simulink model "mcs_ut"  (Simulink 8.1)
settings: Solver=FixedStepDiscrete  StartTime=0.0  StopTime=Inf  FixedStep=0.005  RelTol=1e-3
PostLoadFcn:
  | , if any(exist('dsrtsu_mdlpostloadfcn', 'file') == [2, 3, 6]), try dsrtsu_mdlpostloadfcn('Execute', bdroot); catch fprintf('Error in PostLoadFcn (dsrtsu_mdlpostloadfcn) for model "%s":\n %s\n', bdroot, lasterr); end, end,
libraries: siltestlib x28, idiada_lib x17, mcs x1
settings Model: DSRTSU_INTERNAL_RTI_VER=450  DSRTSU_INTERNAL_RTI_TYPE=rti1401  RTICANMMDATA=struct('GeneralSetupData',struct('modelroot','D:\ELN150201_TAIWAN\trunk\AdasDragon\software\sw_development\arch\app\ifo','generalsettings',struct('filesettings',struct('destfolder',struct('Name','RTICANMM_FILES','Check',1),'buildfolder',struct('Name','.','Check',1),'AbsDestfolder',struct('Name','D:\ELN150201_TAIWAN\trunk\AdasDragon\software\sw_development\arch\app\ifo\RTICANMM_FILES'),'AbsBuildfolder',struct('Name','D:\ELN150201_TAIWAN\trunk\AdasDragon\software\sw_development\arch\app\ifo'))),'options',struct('addpaths',1,'rmpaths',1,'addtrcexclusion',logical(1),'cannavigator',struct('checkmonitoring',0),'show_usrtrc',0,'use_usrtrc',0),'advanced',struct('options',[1 1 1 1 1 1 1 1 1 1 1 1 1 1 1 1 1 1 1 1 1 1 1 1 1 1 1 1 1 1 1 1 1 1 1 1 1 1 1 1 1 1 1 1 1 1 1 1 1 1 1 1 1 1 1 1 1 1 1 1 1 1 1 1 1 1 1 1 1 1 1 1 1 1 1 1 1 1 1 1 1 1 1 1 1 1 1 1 1 1 1 1 1 1 1 1 1 1 1 1]),'MPSetup',{{}},'modelname','mcs_ut','block','mcs_ut'))  DSRTSU_INTERNAL_RTIFPGA=40  Creator=tescamilla  LastModifiedBy=AT015555  BufferReuse=off
settings DataIOCC: SignalLoggingSaveFormat=Dataset
settings OptimizationCC: BlockReduction=off  OptimizeBlockIOStorage=off  BufferReuse=off  ExpressionFolding=off  ExpressionDepthLimit=128  LocalBlockOutputs=off
settings DebuggingCC: FcnCallInpInsideContextMsg=EnableAllAsError
settings HardwareCC: ProdIntDivRoundTo=Zero  ProdEndianess=BigEndian  ProdHWDeviceType=Generic->Custom  TargetIntDivRoundTo=Zero  TargetEndianess=BigEndian  TargetHWDeviceType=Generic->Custom
settings RTWCC: SystemTargetFile=rti1401.tlc  MakeCommand=make_rti  TemplateMakefile=rti1401.tmf  Description=dSPACE DS1401 Hardware Platform  ProcessScript=rti1401_make_rtw_hook
settings STFCustomTargetCC: CodeReplacementLibrary=ANSI_C  ParMdlRefBuildCompliant=on  GeneratePreprocessorConditionals=Disable all  MatFileLogging=on  SystemTargetFile=rti1401.tlc
settings GRTTargetCC: CompOptLevelCompliant=off  ConcurrentExecutionCompliant=off  ExtModeMexFile=noextcomm
settings CustomProperty: DataType=RTWOptions_EnumType_C__Program Files (x86)_dSPACE RCPHIL 2014-B_MATLAB_RTI_RTI1401_TLC_rti1401_1InitialSimState  Value=RUN
settings EnumStrPairs: String=RUN

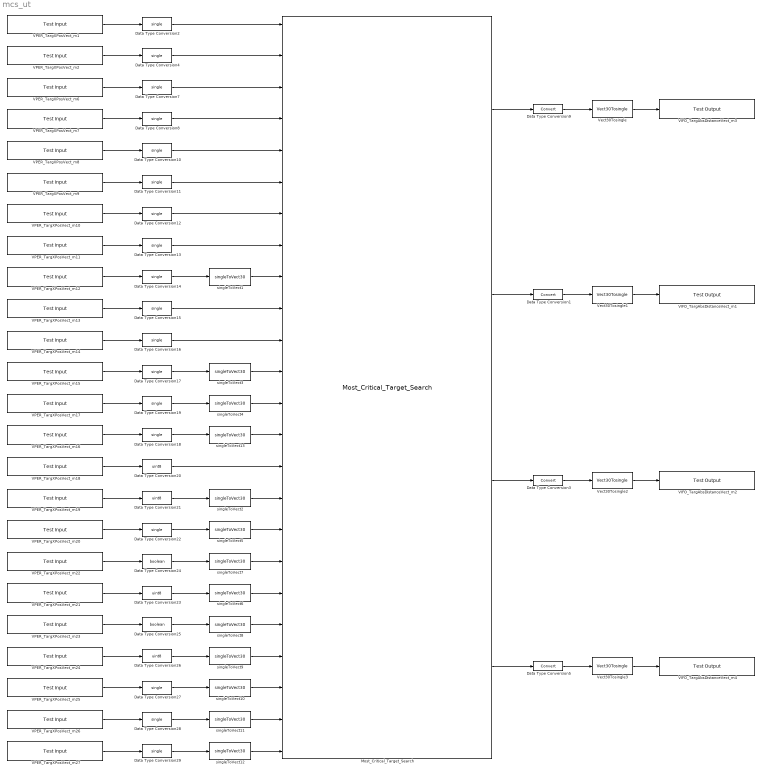
== system mcs_ut ==
  Data Type Conversion{1,3,5,9} (4 alike) : DataTypeConversion
  Data Type Conversion{2,4,7..8,10..19,22,27..29} (18 alike) : DataTypeConversion  OutDataTypeStr=single
  Data Type Conversion{20..21,23,26} (4 alike) : DataTypeConversion  OutDataTypeStr=uint8
  Data Type Conversion24 : DataTypeConversion  OutDataTypeStr=boolean
  Data Type Conversion25 : DataTypeConversion  OutDataTypeStr=boolean
  Most_Critical_Target_Search : mcs/Most_Critical_Target_Search
  VIFO_TargAbsDistanceVect_m1 : siltestlib/Test Output  varname=VIFO_AEBMCTTargId_num  sampletime=-1
  VIFO_TargAbsDistanceVect_m2 : siltestlib/Test Output  varname=VIFO_ACCMCTTargId_num  sampletime=-1
  VIFO_TargAbsDistanceVect_m3 : siltestlib/Test Output  varname=VIFO_FCWMCTTargId_num  sampletime=-1
  VIFO_TargAbsDistanceVect_m4 : siltestlib/Test Output  varname=VIFO_VRUMCTTargId_num  sampletime=-1
  VPER_TargXPosVect_m1 : siltestlib/Test Input  varname=VPER_LaneC0L_m  sampletime=0.005
  VPER_TargXPosVect_m10 : siltestlib/Test Input  varname=VPER_LaneC2R_rat  sampletime=0.005
  VPER_TargXPosVect_m11 : siltestlib/Test Input  varname=VPER_LaneC3R_rat  sampletime=0.005
  VPER_TargXPosVect_m12 : siltestlib/Test Input  varname=VPER_TargIdVect30_m  sampletime=0.005
  VPER_TargXPosVect_m13 : siltestlib/Test Input  varname=VDINR_YawRate_degps  sampletime=0.005
  VPER_TargXPosVect_m14 : siltestlib/Test Input  varname=VDINR_SteerAngle_deg  sampletime=0.005
  VPER_TargXPosVect_m15 : siltestlib/Test Input  varname=VPER_TargVehWidthVect30_m  sampletime=0.005
  VPER_TargXPosVect_m16 : siltestlib/Test Input  varname=VPER_TargYPosVect30_m  sampletime=0.005
  VPER_TargXPosVect_m17 : siltestlib/Test Input  varname=VPER_TargXPosVect30_m  sampletime=0.005
  VPER_TargXPosVect_m18 : siltestlib/Test Input  varname=VPER_NumberOfTargets_enum  sampletime=0.005
  VPER_TargXPosVect_m19 : siltestlib/Test Input  varname=VPER_TargTypeVect30_enum  sampletime=0.005
  VPER_TargXPosVect_m2 : siltestlib/Test Input  varname=VPER_LaneC1L_rad  sampletime=0.005
  VPER_TargXPosVect_m20 : siltestlib/Test Input  varname=VPER_TargExisProbVect30_num  sampletime=0.005
  VPER_TargXPosVect_m21 : siltestlib/Test Input  varname=VPER_RadDynPropertyVect30_enum  sampletime=0.005
  VPER_TargXPosVect_m22 : siltestlib/Test Input  varname=VPER_RadObjValidVect30_flg  sampletime=0.005
  VPER_TargXPosVect_m23 : siltestlib/Test Input  varname=VPER_CamObsValidVect30_flg  sampletime=0.005
  VPER_TargXPosVect_m24 : siltestlib/Test Input  varname=VPER_CamObsStatusVect30_enum  sampletime=0.005
  VPER_TargXPosVect_m25 : siltestlib/Test Input  varname=VIFO_TargAbsSpeedXVect30_mps  sampletime=0.005
  VPER_TargXPosVect_m26 : siltestlib/Test Input  varname=VIFO_TargAbsSpeedYVect30_mps  sampletime=0.005
  VPER_TargXPosVect_m27 : siltestlib/Test Input  varname=VIFO_TargVehRelSpeedXVect30_mps  sampletime=0.005
  VPER_TargXPosVect_m6 : siltestlib/Test Input  varname=VPER_LaneC2L_rat  sampletime=0.005
  VPER_TargXPosVect_m7 : siltestlib/Test Input  varname=VPER_LaneC3L_rat  sampletime=0.005
  VPER_TargXPosVect_m8 : siltestlib/Test Input  varname=VPER_LaneC0R_m  sampletime=0.005
  VPER_TargXPosVect_m9 : siltestlib/Test Input  varname=VPER_LaneC1R_rad  sampletime=0.005
  Vect30Tosingle{,1..3} (4 alike) : idiada_lib/Vect30Tosingle
  singleToVect{1..13} (13 alike) : idiada_lib/singleToVect30
  wires:
  Data Type Conversion9/1 -> Vect30Tosingle/1
  Most_Critical_Target_Search/1 -> Data Type Conversion9/1
  Vect30Tosingle/1 -> VIFO_TargAbsDistanceVect_m3/1
  Data Type Conversion1/1 -> Vect30Tosingle1/1
  Vect30Tosingle1/1 -> VIFO_TargAbsDistanceVect_m1/1
  Most_Critical_Target_Search/2 -> Data Type Conversion1/1
  VPER_TargXPosVect_m1/1 -> Data Type Conversion2/1
  VPER_TargXPosVect_m2/1 -> Data Type Conversion4/1
  VPER_TargXPosVect_m6/1 -> Data Type Conversion7/1
  VPER_TargXPosVect_m7/1 -> Data Type Conversion8/1
  VPER_TargXPosVect_m8/1 -> Data Type Conversion10/1
  VPER_TargXPosVect_m9/1 -> Data Type Conversion11/1
  VPER_TargXPosVect_m10/1 -> Data Type Conversion12/1
  VPER_TargXPosVect_m11/1 -> Data Type Conversion13/1
  Data Type Conversion4/1 -> Most_Critical_Target_Search/2
  Data Type Conversion13/1 -> Most_Critical_Target_Search/8
  Data Type Conversion2/1 -> Most_Critical_Target_Search/1
  Data Type Conversion8/1 -> Most_Critical_Target_Search/4
  Data Type Conversion7/1 -> Most_Critical_Target_Search/3
  Data Type Conversion12/1 -> Most_Critical_Target_Search/7
  Data Type Conversion11/1 -> Most_Critical_Target_Search/6
  Data Type Conversion10/1 -> Most_Critical_Target_Search/5
  VPER_TargXPosVect_m12/1 -> Data Type Conversion14/1
  Data Type Conversion14/1 -> singleToVect1/1
  singleToVect1/1 -> Most_Critical_Target_Search/9
  VPER_TargXPosVect_m13/1 -> Data Type Conversion15/1
  Data Type Conversion15/1 -> Most_Critical_Target_Search/10
  VPER_TargXPosVect_m14/1 -> Data Type Conversion16/1
  Data Type Conversion16/1 -> Most_Critical_Target_Search/11
  VPER_TargXPosVect_m15/1 -> Data Type Conversion17/1
  Data Type Conversion17/1 -> singleToVect3/1
  VPER_TargXPosVect_m16/1 -> Data Type Conversion18/1
  VPER_TargXPosVect_m17/1 -> Data Type Conversion19/1
  VPER_TargXPosVect_m18/1 -> Data Type Conversion20/1
  VPER_TargXPosVect_m19/1 -> Data Type Conversion21/1
  Data Type Conversion21/1 -> singleToVect2/1
  singleToVect2/1 -> Most_Critical_Target_Search/16
  Data Type Conversion20/1 -> Most_Critical_Target_Search/15
  Data Type Conversion19/1 -> singleToVect4/1
  Data Type Conversion18/1 -> singleToVect13/1
  VPER_TargXPosVect_m20/1 -> Data Type Conversion22/1
  Data Type Conversion22/1 -> singleToVect5/1
  singleToVect5/1 -> Most_Critical_Target_Search/17
  VPER_TargXPosVect_m21/1 -> Data Type Conversion23/1
  Data Type Conversion23/1 -> singleToVect6/1
  singleToVect6/1 -> Most_Critical_Target_Search/19
  VPER_TargXPosVect_m22/1 -> Data Type Conversion24/1
  Data Type Conversion24/1 -> singleToVect7/1
  singleToVect7/1 -> Most_Critical_Target_Search/18
  VPER_TargXPosVect_m23/1 -> Data Type Conversion25/1
  Data Type Conversion25/1 -> singleToVect8/1
  singleToVect8/1 -> Most_Critical_Target_Search/20
  VPER_TargXPosVect_m24/1 -> Data Type Conversion26/1
  Data Type Conversion26/1 -> singleToVect9/1
  singleToVect9/1 -> Most_Critical_Target_Search/21
  VPER_TargXPosVect_m25/1 -> Data Type Conversion27/1
  Data Type Conversion27/1 -> singleToVect10/1
  singleToVect10/1 -> Most_Critical_Target_Search/22
  VPER_TargXPosVect_m26/1 -> Data Type Conversion28/1
  Data Type Conversion28/1 -> singleToVect11/1
  singleToVect11/1 -> Most_Critical_Target_Search/23
  VPER_TargXPosVect_m27/1 -> Data Type Conversion29/1
  Data Type Conversion29/1 -> singleToVect12/1
  singleToVect12/1 -> Most_Critical_Target_Search/24
  Data Type Conversion3/1 -> Vect30Tosingle2/1
  Vect30Tosingle2/1 -> VIFO_TargAbsDistanceVect_m2/1
  Most_Critical_Target_Search/3 -> Data Type Conversion3/1
  Data Type Conversion5/1 -> Vect30Tosingle3/1
  Vect30Tosingle3/1 -> VIFO_TargAbsDistanceVect_m4/1
  Most_Critical_Target_Search/4 -> Data Type Conversion5/1
  singleToVect3/1 -> Most_Critical_Target_Search/12
  singleToVect4/1 -> Most_Critical_Target_Search/13
  singleToVect13/1 -> Most_Critical_Target_Search/14
